simulink model "ph_plant"  (Simulink 5.0)
settings: Solver=ode45  SolverMode=SingleTasking  StartTime=0.0  StopTime=10  FixedStep=0.01  RelTol=1e-3  AbsTol=1e-6
PreLoadFcn:
  | setup_ph
libraries: cmlib x6, simulink x1
settings Model: LastModifiedBy=ansgar  ExtModeTrigMode=oneshot  ExtModeArmWhenConnect=off  LimitDataPoints=off  BlockReductionOpt=off  BooleanDataType=off

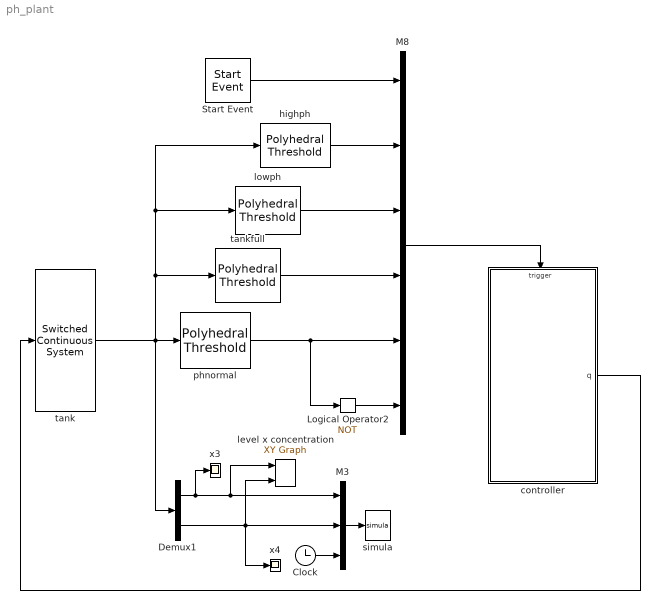
== system ph_plant ==
  Clock : Clock
  Demux1 : Demux  Outputs=2
  Logical Operator2 : Logic  Operator=NOT
  M3 : Mux  Inputs=3
  M8 : Mux  Inputs=6
  Start Event : cmlib/Start Event  steptime=0.0001  initval=0  finival=1  sampletime=0  interpret=on  enable=on
  controller : Stateflow chart  TreatAsAtomicUnit=on
  highph : cmlib/Polyhedral Threshold  polyhedron=highph
  level x concentration : simulink/Sinks/XY Graph  xmin=0  xmax=1  ymin=6.95  ymax=7.25  st=-1
  lowph : cmlib/Polyhedral Threshold  polyhedron=lowph
  phnormal : cmlib/Polyhedral Threshold  polyhedron=phnormal
  simula : ToWorkspace  VariableName=simula  SampleTime=0.01  SaveFormat=Array
  tank : cmlib/Switched Continuous System  AncestorBlock=cmlib/Switched Continuous System  nx=2  use_sd=off  nup=[]  nz=[]  use_reset=off  nu=1  x0=[0; 7.1]  swfunc=PH_function  ICS=PH_ICS  AR=PH_AR  use_param=off  p0=[]  PaCs=[]
  tankfull : cmlib/Polyhedral Threshold  polyhedron=tankfull
  x3 : Scope
      settings: TickLabels=on  TimeRange=12  YMin=0.55  YMax=1.2  DataFormat=Array
  x4 : Scope
      settings: TickLabels=on  TimeRange=10  YMin=7.1  YMax=7.4  DataFormat=Array
  wires:
  M8/1 -> controller/Trigger
  controller/1(q) -> tank/1
  Start Event/1 -> M8/1
  tank/1 -> tankfull/1, lowph/1, highph/1, phnormal/1, Demux1/1
  M3/1 -> simula/1
  Clock/1 -> M3/3
  Demux1/2 -> M3/2, level x concentration/2, x4/1
  Demux1/1 -> M3/1, level x concentration/1, x3/1
  highph/1 -> M8/2
  lowph/1 -> M8/3
  tankfull/1 -> M8/4
  phnormal/1 -> Logical Operator2/1, M8/5
  Logical Operator2/1 -> M8/6

== stateflow chart controller ==
  state normal/
    entry: q=1;
  state avoid/
    entry: q=4;
  state alkaline/
    entry: q=2;
  state acid/
    entry: q=3;
  state reach/
    entry: q=5;
  (default) -> normal : start
  normal -> alkaline : High_pH
  normal -> acid : Low_pH
  alkaline -> normal : pH_not_High
  acid -> normal : pH_not_Low
  acid -> avoid : full
  alkaline -> avoid : full
  normal -> reach : full
  data: q output double
  events: start input RISING_EDGE_EVENT; High_pH input RISING_EDGE_EVENT; Low_pH input RISING_EDGE_EVENT; full input RISING_EDGE_EVENT; pH_not_High input RISING_EDGE_EVENT; pH_not_Low input RISING_EDGE_EVENT
